simulink library "INT_Rail_TempLim"  (R2016b)
settings: Solver=VariableStepAuto  StartTime=0.0  StopTime=10.0  RelTol=1e-3
settings Model: Creator=Administrator  LastModifiedBy=Administrator

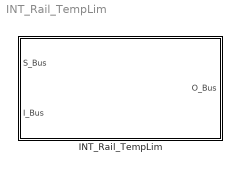
== system INT_Rail_TempLim ==
  INT_Rail_TempLim : Subsystem

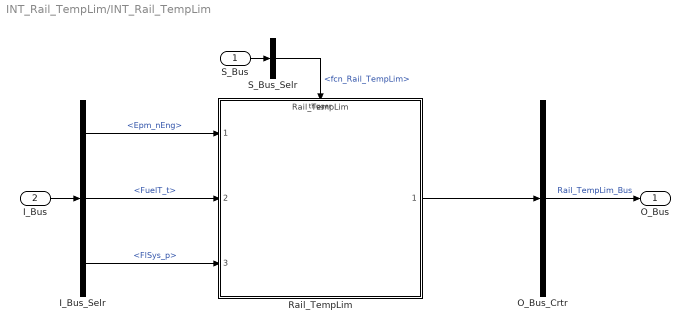
== system INT_Rail_TempLim/INT_Rail_TempLim ==
  S_Bus : Inport
  I_Bus : Inport  Port=2
  I_Bus_Selr : BusSelector  OutputSignals=Epm_nEng,FuelT_t,FlSys_p
  O_Bus_Crtr : BusCreator  Inputs=1
  Rail_TempLim : ModelReference  ModelNameDialog=Rail_TempLim  SimulationMode=Normal  ModelReferenceVersion=1.4  TriggerPortName=function  TriggerPortTriggerType=function-call  TriggerPortStatesWhenEnabling=held
  S_Bus_Selr : BusSelector  OutputSignals=fcn_Rail_TempLim
  O_Bus : Outport
  wires:
  S_Bus_Selr/1 -> Rail_TempLim/Trigger  "<fcn_Rail_TempLim>"
  S_Bus/1 -> S_Bus_Selr/1
  I_Bus/1 -> I_Bus_Selr/1
  I_Bus_Selr/1 -> Rail_TempLim/1  "<Epm_nEng>"
  I_Bus_Selr/2 -> Rail_TempLim/2  "<FuelT_t>"
  I_Bus_Selr/3 -> Rail_TempLim/3  "<FlSys_p>"
  O_Bus_Crtr/1 -> O_Bus/1  "Rail_TempLim_Bus"
  Rail_TempLim/1 -> O_Bus_Crtr/1
